simulink model "momentum_unload_test2"  (R2016b)
settings: Solver=VariableStepAuto  StartTime=0.0  StopTime=5400  MinStep=0.001  RelTol=1e-3
libraries: dynamics_lib x1, environment_lib x1, momentum_dump_lib_test x1, pd_control_lib x1, RW_assembly_simple_lib x1
settings Model: Creator=taylorreynolds  LastModifiedBy=evich

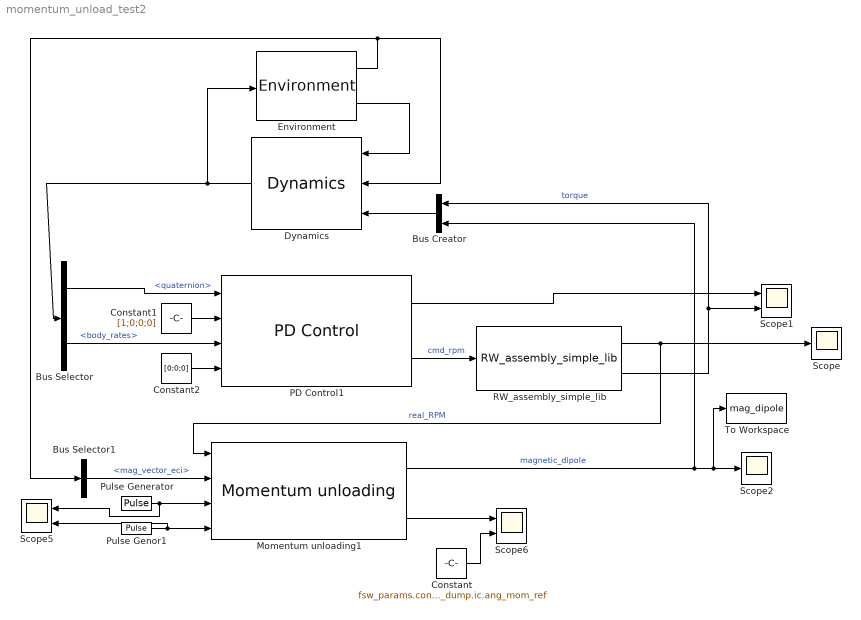
== system momentum_unload_test2 ==
  Bus Creator : BusCreator  Inputs=2
  Bus Selector : BusSelector  OutputSignals=quaternion,body_rates
  Bus Selector1 : BusSelector  OutputSignals=mag_vector_eci
  Constant : Constant  Value=fsw_params.control.p_dump.ic.ang_mom_ref
  Constant1 : Constant  Value=[1;0;0;0]
  Constant2 : Constant  Value=[0;0;0]
  Dynamics : dynamics_lib/Dynamics
  Environment : environment_lib/Environment
  Momentum unloading1 : momentum_dump_lib_test/Momentum unloading
  PD Control1 : pd_control_lib/PD Control
  Pulse Generator : DiscretePulseGenerator  PulseType=Time based  Period=fsw_params.actuators.ppt.sync_pulse  PulseWidth=fsw_params.actuators.ppt.t_charge_pct
  Pulse Genor1 : DiscretePulseGenerator  PulseType=Time based  Period=10  PulseWidth=sim_params.sensors.magnetometer.valid_pct
  RW_assembly_simple_lib : RW_assembly_simple_lib/RW_assembly_simple_lib  natural_frequency=100  damping_ratio=1  max_rate=100
  Scope : Scope
  Scope1 : Scope  NumInputPorts=2
  Scope2 : Scope
  Scope5 : Scope  NumInputPorts=2
  Scope6 : Scope  NumInputPorts=2
  To Workspace : ToWorkspace  VariableName=mag_dipole  SaveFormat=Timeseries  SampleTime=-1
  wires:
  Environment/2 -> Dynamics/1
  Environment/1 -> Dynamics/2, Bus Selector1/1
  Dynamics/1 -> Environment/1, Bus Selector/1
  Bus Selector/2 -> PD Control1/3  "<body_rates>"
  Bus Selector/1 -> PD Control1/1  "<quaternion>"
  Bus Creator/1 -> Dynamics/3
  Momentum unloading1/1 -> Bus Creator/2, To Workspace/1, Scope2/1  "magnetic_dipole"
  PD Control1/2 -> RW_assembly_simple_lib/1  "cmd_rpm"
  RW_assembly_simple_lib/2 -> Bus Creator/1, Scope1/2  "torque"
  RW_assembly_simple_lib/1 -> Momentum unloading1/1, Scope/1  "real_RPM"
  Bus Selector1/1 -> Momentum unloading1/2  "<mag_vector_eci>"
  Pulse Generator/1 -> Momentum unloading1/3, Scope5/1
  Pulse Genor1/1 -> Momentum unloading1/4, Scope5/2
  Momentum unloading1/2 -> Scope6/1
  PD Control1/1 -> Scope1/1
  Constant1/1 -> PD Control1/2
  Constant2/1 -> PD Control1/4
  Constant/1 -> Scope6/2
